simulink model "meart_target_60"  (Simulink 6.5)
settings: Solver=FixedStepDiscrete  StartTime=0.0  StopTime=Inf  FixedStep=0.0005  RelTol=1e-3
values from neighbouring files (symbols this model uses):
  channelmask = ones(1,60)    [run_experiment.m]
  offset = mean(data)    [setthresh.m]
  stimcombs = [I; zeros(60)]    [run_experiment.m]
  stimtimes = (cumsum(dstimtimes)+T_start)*2000    [run_experiment.m]
  stimulusintensity = [400 500 600 700 800]    [run_experiment.m]
  switchtimes = []    [run_experiment.m]
  synctimes = 0    [run_experiment.m]
  threshold = -10*std(data)    [setthresh.m]
undefined symbols (not defined in the file or in its folder): MF, onsetchannelmask, PD2
libraries: simulink x24, meaworklibrary x16, xpclib x9, dspstat3 x2, xpcueilib x2, dspindex x1, dspbuff3 x1, dspsigops x1
(part 2 of 2)

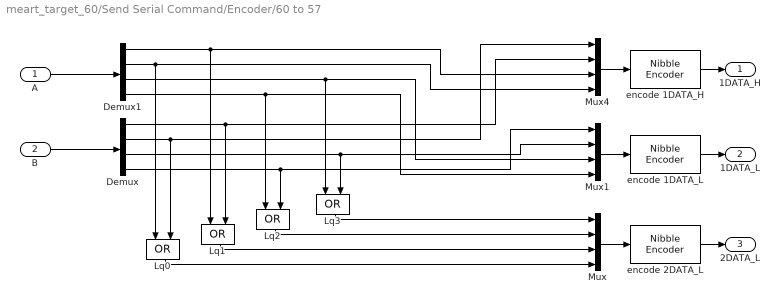
== system meart_target_60/Send Serial Command/Encoder/60 to 57 ==
  A : Inport  PortDimensions=4
  B : Inport  Port=2  PortDimensions=4
  Demux : Demux
  Demux1 : Demux
  Lq{0..3} (4 alike) : Logic  Orientation=down  Operator=OR  AllPortsSameDT=off  OutDataTypeMode=Specify via dialog
  Mux : Mux
  Mux1 : Mux
  Mux4 : Mux
  encode 1DATA_H : meaworklibrary/Nibble Encoder  SystemSampleTime=-1
  encode 1DATA_L : meaworklibrary/Nibble Encoder  SystemSampleTime=-1
  encode 2DATA_L : meaworklibrary/Nibble Encoder  SystemSampleTime=-1
  1DATA_H : Outport  DataType=uint8
  1DATA_L : Outport  Port=2  DataType=uint8
  2DATA_L : Outport  Port=3  DataType=uint8
  wires:
  B/1 -> Demux/1
  A/1 -> Demux1/1
  Mux4/1 -> encode 1DATA_H/1
  encode 1DATA_H/1 -> 1DATA_H/1
  Mux1/1 -> encode 1DATA_L/1
  encode 1DATA_L/1 -> 1DATA_L/1
  Demux1/1 -> Mux4/3, Lq1/1
  Demux/1 -> Mux4/2, Lq1/2
  Demux1/2 -> Mux4/4, Lq0/1
  Demux/2 -> Mux4/1, Lq0/2
  Demux1/3 -> Mux1/3, Lq3/1
  Demux/3 -> Mux1/2, Lq3/2
  Demux1/4 -> Mux1/4, Lq2/1
  Demux/4 -> Mux1/1, Lq2/2
  Mux/1 -> encode 2DATA_L/1
  encode 2DATA_L/1 -> 2DATA_L/1
  Lq3/1 -> Mux/1
  Lq2/1 -> Mux/2
  Lq1/1 -> Mux/3
  Lq0/1 -> Mux/4

== system meart_target_60/DAQ Frame (8-sample)/Burst Detection/Burst Refractory/Triggered Disable ==
  Trigger : Inport  DataType=boolean
  " Zero" : simulink/Logic and Bit Operations/Compare To Zero  SystemSampleTime=-1  relop===  LogicOutDataTypeMode=boolean  ZeroCross=off
  At Zero : simulink/Logic and Bit Operations/Compare To Zero  Orientation=left  SystemSampleTime=-1  relop===  LogicOutDataTypeMode=boolean  ZeroCross=off
  Constant : Constant  Value=holdtimesamples  OutDataTypeMode=uint32  OutDataType=sfix(16)  ConRadixGroup=Use specified scaling  OutScaling=2^0  SampleTime=inf  FramePeriod=inf
  Count down : Constant  Value=1  OutDataTypeMode=boolean  OutDataType=sfix(16)  ConRadixGroup=Use specified scaling  OutScaling=2^0  SampleTime=inf  FramePeriod=inf
  Count down Disable : Logic  Operator=NAND  AllPortsSameDT=off  OutDataTypeMode=Specify via dialog
  Logical Operator : Logic  AllPortsSameDT=off  OutDataTypeMode=Boolean
  Sum : Sum  Inputs=|-+  OutDataTypeMode=uint32
  Switch : Switch  Criteria=u2 > Threshold
  Unit Delay : UnitDelay  Orientation=left  SampleTime=-1
  Enable : Outport
  wires:
  Constant/1 -> Switch/1
  Switch/1 -> " Zero"/1, Unit Delay/1
  Unit Delay/1 -> At Zero/1, Sum/2
  Logical Operator/1 -> Switch/2
  At Zero/1 -> Logical Operator/2, Count down Disable/2
  Sum/1 -> Switch/3
  Count down Disable/1 -> Sum/1
  Count down/1 -> Count down Disable/1
  Trigger/1 -> Logical Operator/1
  " Zero"/1 -> Enable/1

== matlab function Network Transmit /UDP Buffered Packet Send/Transmit Logic ==
  data: send_packet output inherited; rcv_sync input uint32; rcv_valid input double; packsize input inherited; send_sync output uint32; dv input boolean; ack output boolean
function [send_packet,send_sync,ack]  =  fcn(rcv_sync,rcv_valid,packsize,dv)
% Transmit Synchronization logic - State controller for the Target application 
%   that controls transmission of a contigyous stream of data from to the host.
%
%   Acknowledge
%
%SYC_RESEND -  This value defines how many cycles to wait for an ACK before 
%  re-transmitting a packet.  The actual resend period is an integer multiple 
%  of the sample period of this block. 
%  Recommendation - it should > 1 and less than the packet size.  
%  If your packet size is 100, I'd recommend a value of around 20.  But the optimum value will
%  depend on many factors, such as sample period, network loading, 
%  network bandwidth, host loading, host latency etc.  
%
% States - 
%  WAIT_DV(0) - This is our initial state and means we're waiting for our
%    a packet to be ready for transmission.  In this state, we ignore all
%    received stuff and simply wait for a complete packet to be ready.  
%
%  WAIT_ACK(1) - Waiting for an acknowledgement.
%
persistent timer;
persistent sync; 
persistent state;

% How many time steps should we wait before re-transmitting a packet?  If this
% value is too small, we can reduce overall channel bandwidth by sending unncessary
% copies of the same data.  If it is too large, we risk overflowing the FIFO due
% to a temporary network blockage.  
% Empirically, this 
% Initialization
syc_resend = double(packsize./2);

if isempty(state),
    state = 1;
    sync = 1;  
    timer = 0;
end
% Waiting for first packet to be ready to go!
%  In this mode, we ignore all received data.  
%  Don't bother with timer, (nothing to resend).  
switch state,
case 1,  % WAIT_DV
    if dv,    % Still waiting!
        timer = 0;
        send_sync = uint32(sync);
        send_packet = 1;
        ack = logical(0);
        state = 2;
    else % Data is ready, send it and move to the next state...        
        send_sync = uint32(0);
        send_packet = 0;
        ack = logical(0);        
    end
otherwise 
%case 2,  % WAIT_ACK
    if (rcv_valid == 1) && (sync == rcv_sync), %Got an ack, and it's correct !!!  
        % I can't send anything on this cycle, because I'm still holding
        %  the previous value
        sync = sync + 1;  % move to the next sync integer
        send_sync = uint32(0);
        send_packet = 0;
        ack = logical(1);
        state = 1;
    else % Still waiting of a valid ack
       timer = timer + 1;
       if timer >= syc_resend,
            send_sync = uint32(sync);  % resend the same sync/data...
            send_packet = 1;
            ack = logical(0);
            timer = 0;
       else 
            send_sync = uint32(0);
            send_packet = 0;
            ack = logical(0);
       end
    end
end
